simulink library "adc_lib"  (R2022b)
settings: Solver=VariableStepAuto  StartTime=0.0  StopTime=10.0  RelTol=1e-3
undefined symbols (not defined in the file): raptor_xcp_function
libraries: Raptor_lib x5, simulink_extras x1
settings Model: Creator=serga  LastModifiedBy=serga

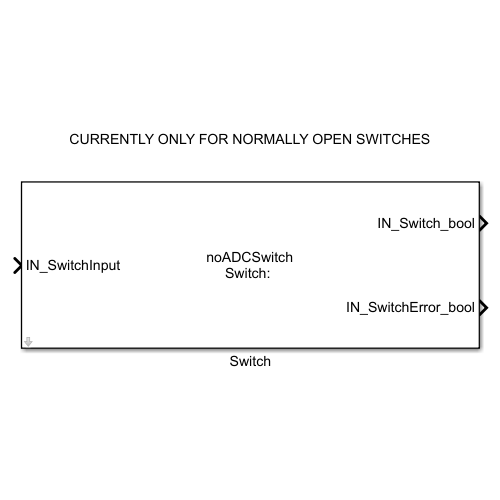
[thumbnail: Simulink's stored preview of the top-level diagram]
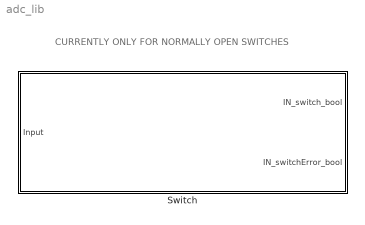
== system adc_lib ==
  note: CURRENTLY ONLY FOR NORMALLY OPEN SWITCHES
  Switch : Subsystem  mask{pos=''}
      mask prompts: pos "Name"
      mask Display:
      | disp(['noADCSwitch\n'...
      |     'Switch: ' pos]);
      | port_label('input', 1, ['IN_' pos 'SwitchInput']);
      | port_label('output', 1, ['IN_' pos 'Switch_bool']);
      | port_label('output', 2, ['IN_' pos 'SwitchError_bool']);

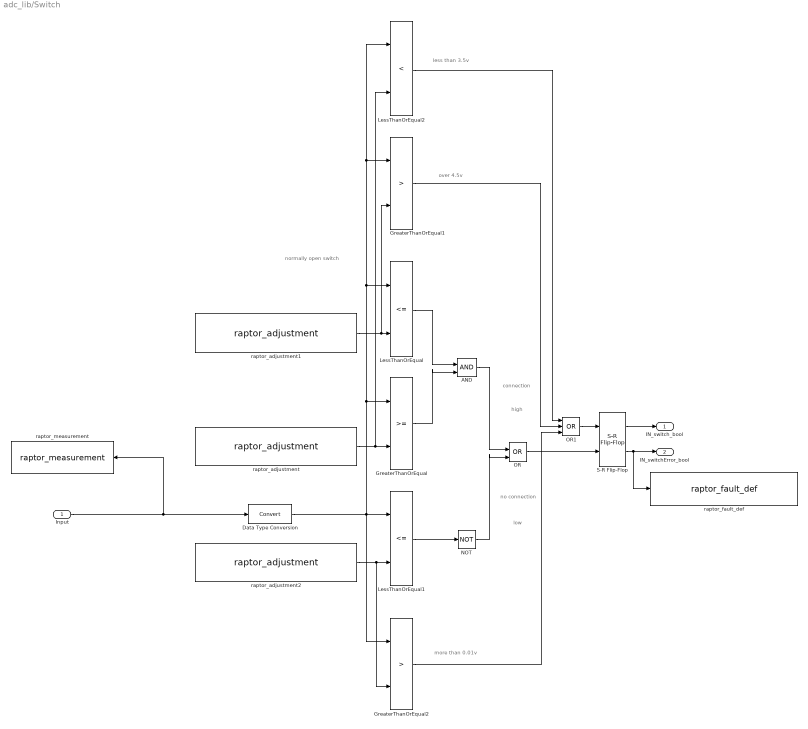
== system adc_lib/Switch ==
  note: more than 0.01v
  note: less than 3.5v
  note: over 4.5v
  note: no connection
  note: connection
  note: high
  note: low
  note: normally open switch
  Input : Inport
  AND : Logic  IconShape=distinctive  AllPortsSameDT=off  OutDataTypeStr=boolean
  Data Type Conversion : DataTypeConversion  SaturateOnIntegerOverflow=off  RndMeth=Floor
  GreaterThanOrEqual : RelationalOperator  OutDataTypeStr=boolean  RndMeth=Simplest  InputSameDT=off
  GreaterThanOrEqual1 : RelationalOperator  Operator=>  OutDataTypeStr=boolean  RndMeth=Simplest  InputSameDT=off
  GreaterThanOrEqual2 : RelationalOperator  Operator=>  OutDataTypeStr=boolean  RndMeth=Simplest  InputSameDT=off
  LessThanOrEqual : RelationalOperator  Operator=<=  OutDataTypeStr=boolean  RndMeth=Simplest  InputSameDT=off
  LessThanOrEqual1 : RelationalOperator  Operator=<=  OutDataTypeStr=boolean  RndMeth=Simplest  InputSameDT=off
  LessThanOrEqual2 : RelationalOperator  Operator=<  OutDataTypeStr=boolean  RndMeth=Simplest  InputSameDT=off
  NOT : Logic  Operator=NOT  IconShape=distinctive  AllPortsSameDT=off  OutDataTypeStr=boolean
  OR : Logic  Operator=OR  IconShape=distinctive  AllPortsSameDT=off  OutDataTypeStr=boolean
  OR1 : Logic  Operator=OR  Inputs=3  IconShape=distinctive  AllPortsSameDT=off  OutDataTypeStr=boolean
  S-R Flip-Flop : simulink_extras/Flip Flops/S-R Flip-Flop  initial_condition=0
  raptor_adjustment : Raptor_lib/Data Storage/raptor_adjustment  paramName=['IN_' pos 'SwitchNOHighUpperThresh']  nameSource=Parameter  initValue=3.5  dataType=double  storage=Calibration  calDispType=Number  calEnum={'False', 'True'}  calGain=1.0  calOffset=0.0  calMax=inf  calMin=-inf  calFormat='-1'  calUnit=''  calHelp=''  calAccess=1  calFunction=raptor_xcp_function(gcb)  calDispHeaders=off  calColHeaders={'Col1' 'Col2' 'Col3'}  calRowHeaders={'Row1' 'Row2' 'Row3'}
      settings: SourceProductName=Raptor
  raptor_adjustment1 : Raptor_lib/Data Storage/raptor_adjustment  paramName=['IN_' pos 'SwitchNOHighLowerThresh']  nameSource=Parameter  initValue=4.5  dataType=double  storage=Calibration  calDispType=Number  calEnum={'False', 'True'}  calGain=1.0  calOffset=0.0  calMax=inf  calMin=-inf  calFormat='-1'  calUnit=''  calHelp=''  calAccess=1  calFunction=raptor_xcp_function(gcb)  calDispHeaders=off  calColHeaders={'Col1' 'Col2' 'Col3'}  calRowHeaders={'Row1' 'Row2' 'Row3'}
      settings: SourceProductName=Raptor
  raptor_adjustment2 : Raptor_lib/Data Storage/raptor_adjustment  paramName=['IN_' pos 'SwitchNOLowLowerThresh']  nameSource=Parameter  initValue=0.01  dataType=double  storage=Calibration  calDispType=Number  calEnum={'False', 'True'}  calGain=1.0  calOffset=0.0  calMax=inf  calMin=-inf  calFormat='-1'  calUnit=''  calHelp=''  calAccess=1  calFunction=raptor_xcp_function(gcb)  calDispHeaders=off  calColHeaders={'Col1' 'Col2' 'Col3'}  calRowHeaders={'Row1' 'Row2' 'Row3'}
      settings: SourceProductName=Raptor
  raptor_fault_def : Raptor_lib/Faults/raptor_fault_def  faultName=['IN_' pos 'SwitchVError_bool']  persist=off  sticky=off  emisRelated=off  singleTrip=off  clearMethod=Standard  xLimit=25  yLimit=50  calEnable=on  addDisable=off  calAccess=1  calFunction='System | FaultManager'
      settings: SourceProductName=Raptor
  raptor_measurement : Raptor_lib/Data Storage/raptor_measurement  paramName=['IN_' pos 'SwitchSig_v']  nameSource=Parameter  calDispType=Number  calEnum={'False', 'True'}  calGain=1.0  calOffset=0.0  calMax=inf  calMin=-inf  calFormat='-1'  calUnit=''  calHelp=''  calAccess=1  calFunction=raptor_xcp_function(gcb)  calVisible=on
      settings: SourceProductName=Raptor
  IN_switch_bool : Outport
  IN_switchError_bool : Outport  Port=2
  wires:
  Input/1 -> raptor_measurement/1, Data Type Conversion/1
  Data Type Conversion/1 -> GreaterThanOrEqual2/1, LessThanOrEqual1/1, LessThanOrEqual2/1, GreaterThanOrEqual1/1, LessThanOrEqual/1, GreaterThanOrEqual/1
  raptor_adjustment/1 -> LessThanOrEqual2/2, GreaterThanOrEqual/2
  raptor_adjustment1/1 -> GreaterThanOrEqual1/2, LessThanOrEqual/2
  raptor_adjustment2/1 -> GreaterThanOrEqual2/2, LessThanOrEqual1/2
  LessThanOrEqual/1 -> AND/1
  GreaterThanOrEqual/1 -> AND/2
  LessThanOrEqual1/1 -> NOT/1
  AND/1 -> OR/1
  NOT/1 -> OR/2
  LessThanOrEqual2/1 -> OR1/1
  GreaterThanOrEqual2/1 -> OR1/3
  OR/1 -> S-R Flip-Flop/2
  S-R Flip-Flop/1 -> IN_switch_bool/1
  OR1/1 -> S-R Flip-Flop/1
  GreaterThanOrEqual1/1 -> OR1/2
  S-R Flip-Flop/2 -> raptor_fault_def/1, IN_switchError_bool/1
